simulink model "testFrame_CalcSpeednDir"  (R2020b)
settings: Solver=FixedStepDiscrete  StartTime=0.0  StopTime=27  FixedStep=200e-6  RelTol=1e-3
libraries: simulink x1
settings Model: DataDictionary=CalcSpeednDir.sldd  NumberOfSteps=500  SnapshotBufferSize=500  SnapshotInterval=100  PacingRate=0.010000  Creator=unix  LastModifiedBy=unix

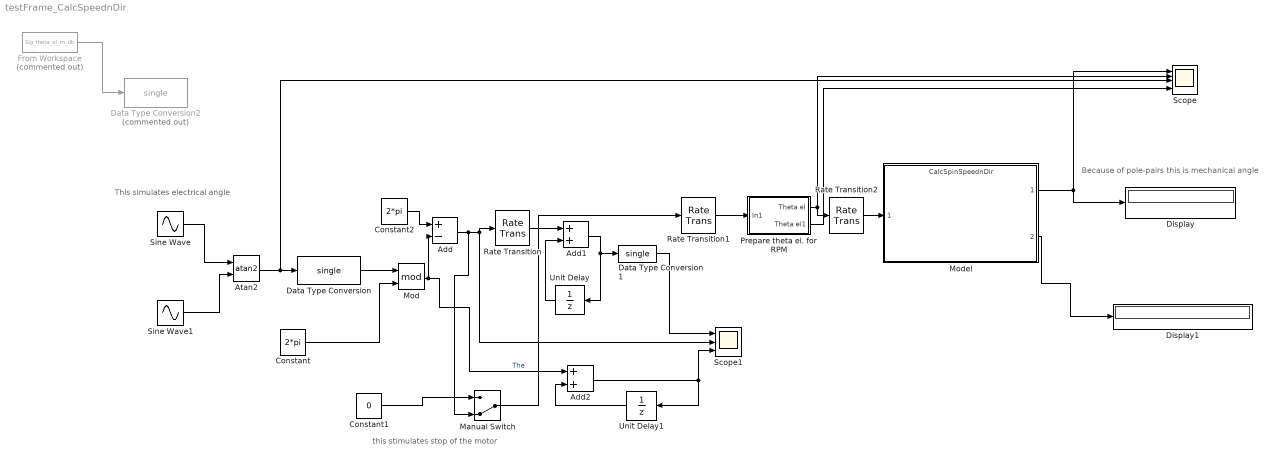
== system testFrame_CalcSpeednDir ==
  note: this stimulates stop of the motor
  note: Because of pole-pairs this is mechanical angle
  note: This simulates electrical angle
  Add : Sum  Inputs=+-
  Add1 : Sum
  Add2 : Sum
  Atan2 : Trigonometry  Operator=atan2
  Constant : Constant  Value=2*pi  OutDataTypeStr=single
  Constant1 : Constant  Value=0  OutDataTypeStr=single
  Constant2 : Constant  Value=2*pi  OutDataTypeStr=Inherit: Inherit via back propagation
  Data Type Conversion : DataTypeConversion  OutDataTypeStr=single
  Data Type Conversion1 : DataTypeConversion  OutDataTypeStr=single
  Data Type Conversion2 : DataTypeConversion  Commented=on  OutDataTypeStr=single
  Display : Display
  Display1 : Display
  From Workspace : FromWorkspace  Commented=on  VariableName=Sig_theta_el_m_db  OutputAfterFinalValue=Holding final value
  Manual Switch : ManualSwitch  CurrentSetting=0
  Mod : Math  Operator=mod  SaturateOnIntegerOverflow=on
  Model : ModelReference  ModelNameDialog=CalcSpinSpeednDir.slx  CachedPortDiscreteRates=[-1]  ModelReferenceVersion=3.13
  Prepare theta el. for RPM : Subsystem
  Rate Transition : RateTransition
  Rate Transition1 : RateTransition
  Rate Transition2 : RateTransition
  Scope : Scope  NumInputPorts=5
  Scope1 : Scope  NumInputPorts=3
  Sine Wave : Sin  Frequency=50  SampleTime=0
  Sine Wave1 : Sin  Frequency=50  Phase=pi/2  SampleTime=0
  Unit Delay : UnitDelay  SampleTime=-1  HasFrameUpgradeWarning=on
  Unit Delay1 : UnitDelay  SampleTime=-1  HasFrameUpgradeWarning=on
  wires:
  Sine Wave/1 -> Atan2/1
  Sine Wave1/1 -> Atan2/2
  Atan2/1 -> Scope/3, Data Type Conversion/1
  Data Type Conversion/1 -> Mod/1
  Constant/1 -> Mod/2
  Model/1 -> Display/1, Scope/1
  Model/2 -> Display1/1
  Constant2/1 -> Add/1
  Mod/1 -> Add/2, Add2/1  "The"
  Constant1/1 -> Manual Switch/1
  Rate Transition/1 -> Add1/1
  Data Type Conversion1/1 -> Scope1/1
  From Workspace/1 -> Data Type Conversion2/1
  Add1/1 -> Unit Delay/1, Data Type Conversion1/1
  Unit Delay/1 -> Add1/2
  Add/1 -> Manual Switch/2, Scope1/2, Rate Transition/1
  Add2/1 -> Scope1/3, Unit Delay1/1
  Unit Delay1/1 -> Add2/2
  Manual Switch/1 -> Rate Transition1/1
  Prepare theta el. for RPM/1(Theta el) -> Rate Transition2/1, Scope/2
  Rate Transition1/1 -> Prepare theta el. for RPM/1(In1)
  Rate Transition2/1 -> Model/1
  Prepare theta el. for RPM/2(Theta el1) -> Scope/5

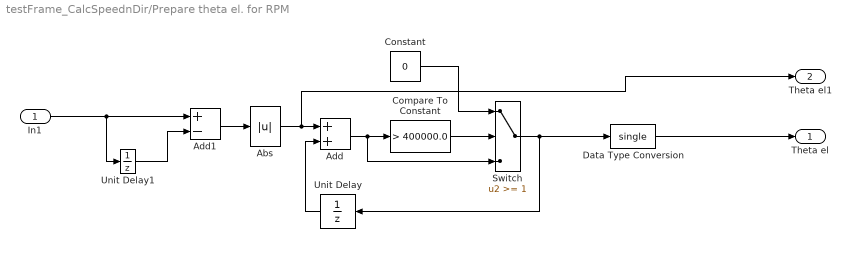
== system testFrame_CalcSpeednDir/Prepare theta el. for RPM ==
  In1 : Inport
  Abs : Abs
  Add : Sum
  Add1 : Sum  Inputs=+-
  Compare To Constant : simulink/Logic and Bit Operations/Compare To Constant  relop=>  const=400000.0  OutDataTypeStr=boolean
  Constant : Constant  Value=0  OutDataTypeStr=single
  Data Type Conversion : DataTypeConversion  OutDataTypeStr=single
  Switch : Switch  Threshold=1  OutDataTypeStr=single
  Unit Delay : UnitDelay  SampleTime=-1  HasFrameUpgradeWarning=on
  Unit Delay1 : UnitDelay  SampleTime=-1  HasFrameUpgradeWarning=on
  Theta el : Outport
  Theta el1 : Outport  Port=2
  wires:
  Unit Delay/1 -> Add/2
  Switch/1 -> Unit Delay/1, Data Type Conversion/1
  In1/1 -> Unit Delay1/1, Add1/1
  Data Type Conversion/1 -> Theta el/1
  Add/1 -> Switch/3, Compare To Constant/1
  Compare To Constant/1 -> Switch/2
  Constant/1 -> Switch/1
  Unit Delay1/1 -> Add1/2
  Add1/1 -> Abs/1
  Abs/1 -> Theta el1/1, Add/1
